simulink model "DSPequivalent"  (R2018b)
settings: Solver=ode5  StartTime=0.0  StopTime=10*R*C  FixedStep=Tsim  RelTol=1e-3
values from neighbouring files (symbols this model uses):
  C = 60e-9    (= 6e-08)    [init_DSPeq.m]
  E = 3.3    [init_DSPeq.m]
  Ki = 0.2/ur    (= 0.1)    [init_DSPeq.m]
  Kp = 1.8    [init_DSPeq.m]
  Nos = 16    [init_DSPeq.m]
  R = 9.8e3    (= 9800)    [init_DSPeq.m]
  Rp = 50e3    (= 50000)    [init_DSPeq.m]
  TBPRD = (round(Tadc/(2*Ttbclk))-1)*ur    [init_DSPeq.m]
  Tpwm = 1/10e3    (= 0.0001)    [init_DSPeq.m]
  Ts = 50e-6    (= 5e-05)    [badnwidth.m]    (also in init_DSPeq.m)
  ur = 2    [init_DSPeq.m]
  Vref1 = 0    [init_DSPeq.m]
  Vref2 = 1    [init_DSPeq.m]
libraries: simulink x4
settings Model: Creator=ruzic  LastModifiedBy=ruzic

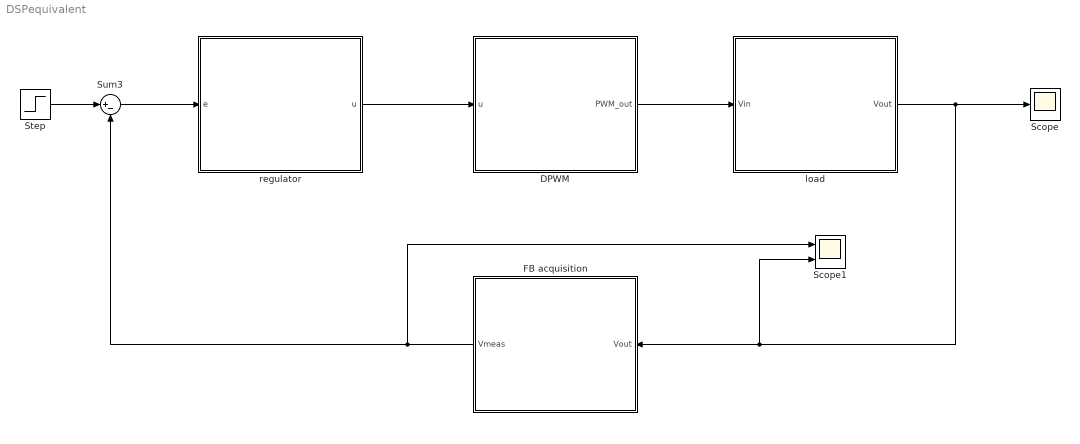
== system DSPequivalent ==
  DPWM : Subsystem
  FB acquisition : Subsystem
  Scope : Scope
  Scope1 : Scope  NumInputPorts=2
  Step : Step  Time=0  Before=Vref1  After=Vref2  SampleTime=Ts
  Sum3 : Sum  Inputs=|+-
  load : Subsystem
  regulator : Subsystem
  wires:
  Sum3/1 -> regulator/1(e)
  Step/1 -> Sum3/1
  DPWM/1(PWM_out) -> load/1(Vin)
  load/1(Vout) -> Scope1/2, FB acquisition/1(Vout), Scope/1
  FB acquisition/1("Vmeas ") -> Scope1/1, Sum3/2
  regulator/1(u) -> DPWM/1(u)

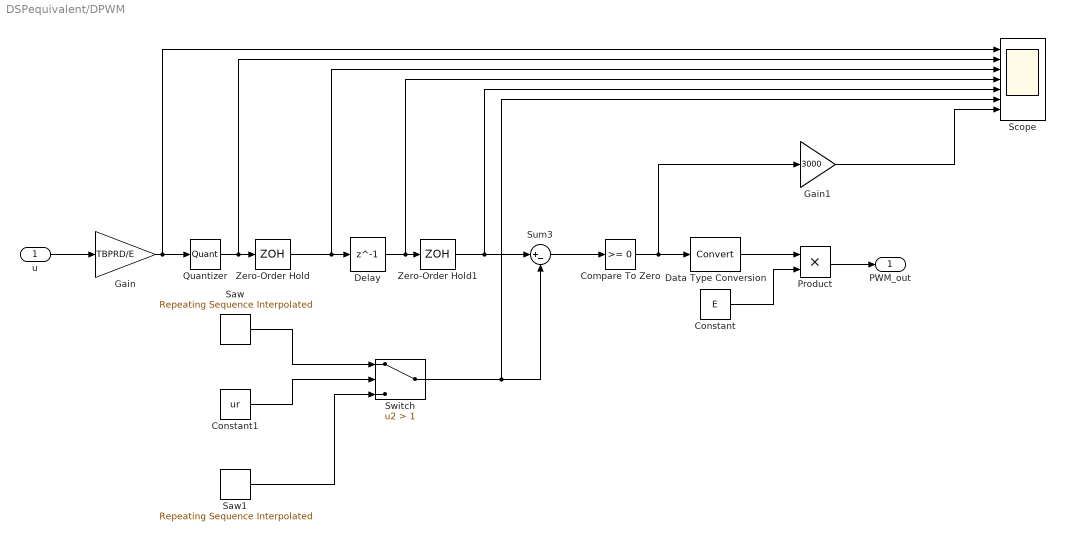
== system DSPequivalent/DPWM ==
  u : Inport
  Compare To Zero : simulink/Logic and Bit Operations/Compare To Zero  relop=>=  OutDataTypeStr=uint8
  Constant : Constant  Value=E
  Constant1 : Constant  Value=ur
  Data Type Conversion : DataTypeConversion
  Delay : Delay  DelayLength=1
  Gain : Gain  Gain=TBPRD/E
  Gain1 : Gain  Gain=3000
  Product : Product
  Quantizer : Quantizer  QuantizationInterval=1
  Saw : simulink/Sources/Repeating Sequence Interpolated  OutValues=TBPRD*[0.5 1 0.5 0 0.5].'  TimeValues=Tpwm/2*[0 0.5 1 1.5 2].'  LookUpMeth=Interpolation-Use End Values  tsamp=Ttbclk  OutMin=[]  OutMax=[]  OutDataTypeStr=double  OutputDataTypeScalingMode=double  OutDataType=fixdt(0,8)  OutScaling=2^-10
  Saw1 : simulink/Sources/Repeating Sequence Interpolated  OutValues=TBPRD*[1 0.5 0 0.5 1].'  TimeValues=Tpwm/2*[0 0.5 1 1.5 2].'  LookUpMeth=Interpolation-Use End Values  tsamp=Ttbclk  OutMin=[]  OutMax=[]  OutDataTypeStr=double  OutputDataTypeScalingMode=double  OutDataType=fixdt(0,8)  OutScaling=2^-10
  Scope : Scope  NumInputPorts=7
  Sum3 : Sum  Inputs=|+-
  Switch : Switch  Criteria=u2 > Threshold  Threshold=1
  Zero-Order Hold : ZeroOrderHold  SampleTime=Ts/2
  Zero-Order Hold1 : ZeroOrderHold  SampleTime=Ts/2
  PWM_out : Outport
  wires:
  u/1 -> Gain/1
  Gain/1 -> Scope/1, Quantizer/1
  Compare To Zero/1 -> Gain1/1, Data Type Conversion/1
  Constant/1 -> Product/2
  Data Type Conversion/1 -> Product/1
  Product/1 -> PWM_out/1
  Quantizer/1 -> Zero-Order Hold/1, Scope/2
  Gain1/1 -> Scope/7
  Sum3/1 -> Compare To Zero/1
  Zero-Order Hold/1 -> Scope/3, Delay/1
  Delay/1 -> Scope/4, Zero-Order Hold1/1
  Zero-Order Hold1/1 -> Scope/5, Sum3/1
  Switch/1 -> Scope/6, Sum3/2
  Saw/1 -> Switch/1
  Constant1/1 -> Switch/2
  Saw1/1 -> Switch/3

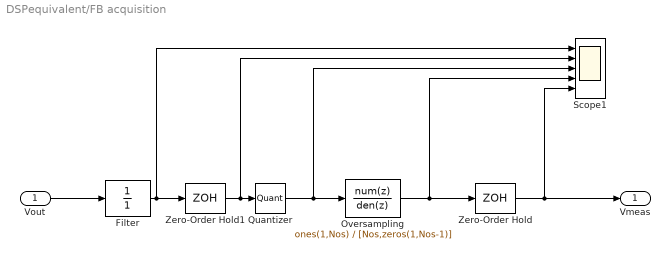
== system DSPequivalent/FB acquisition ==
  Vout : Inport
  Filter : TransferFcn  Denominator=[1]
  Oversampling : DiscreteTransferFcn  Numerator=ones(1,Nos)  Denominator=[Nos,zeros(1,Nos-1)]
  Quantizer : Quantizer  QuantizationInterval=3.1/2^12
  Scope1 : Scope  NumInputPorts=5
  Zero-Order Hold : ZeroOrderHold  SampleTime=Ts
  Zero-Order Hold1 : ZeroOrderHold  SampleTime=Tpwm/Nos
  "Vmeas " : Outport
  wires:
  Zero-Order Hold1/1 -> Scope1/2, Quantizer/1
  Oversampling/1 -> Scope1/4, Zero-Order Hold/1
  Filter/1 -> Scope1/1, Zero-Order Hold1/1
  Vout/1 -> Filter/1
  Quantizer/1 -> Scope1/3, Oversampling/1
  Zero-Order Hold/1 -> Scope1/5, "Vmeas "/1

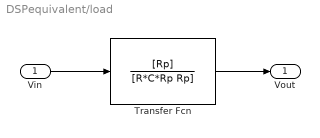
== system DSPequivalent/load ==
  Vin : Inport
  Transfer Fcn : TransferFcn  Numerator=[Rp]  Denominator=[R*C*Rp Rp]
  Vout : Outport
  wires:
  Vin/1 -> Transfer Fcn/1
  Transfer Fcn/1 -> Vout/1

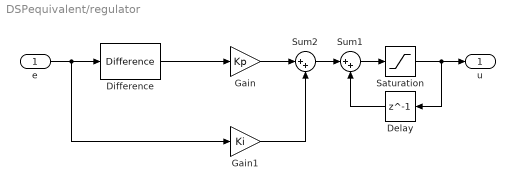
== system DSPequivalent/regulator ==
  e : Inport
  Delay : Delay  DelayLength=1
  Difference : simulink/Discrete/Difference  ICPrevInput=0.0  OutMin=[]  OutMax=[]  OutDataType=fixdt(1, 16)  OutScaling=2^-10  DoSatur=off
  Gain : Gain  Gain=Kp
  Gain1 : Gain  Gain=Ki
  Saturation : Saturate  UpperLimit=E  LowerLimit=0
  Sum1 : Sum  Inputs=|++
  Sum2 : Sum  Inputs=|++
  u : Outport
  wires:
  Sum1/1 -> Saturation/1
  Saturation/1 -> Delay/1, u/1
  Sum2/1 -> Sum1/1
  Delay/1 -> Sum1/2
  Gain/1 -> Sum2/1
  Gain1/1 -> Sum2/2
  Difference/1 -> Gain/1
  e/1 -> Gain1/1, Difference/1
